simulink model "etc_plant_tf"  (R2022b)
settings: Solver=VariableStepAuto  StartTime=0.0  StopTime=20  RelTol=1e-3  EnableMultiTasking=on
PreLoadFcn:
  | % Throttle body parameters
  | etc_plant_data;
  | 
  | % Input data
  | load throttle_input;
values from neighbouring files (symbols this model uses):
  J = 2.45e-4    (= 0.000245)    [etc_plant_data.m]
  Kd = 0.03    [etc_plant_data.m]
  Km = 3.0    (= 3)    [etc_plant_data.m]
  Ks = 0.2    [etc_plant_data.m]
  theta_eq = pi/6    (= 0.523598775598)    [etc_plant_data.m]
settings Model: Creator=nicholas  LastModifiedBy=bensweet
settings SolverCC: ZeroCrossControl=EnableAll  AlgebraicLoopSolver=TrustRegion  AutoInsertRateTranBlk=on
settings DataIOCC: ExternalInput=[t, duty, direction]  LoadExternalInput=on  SaveState=on  ReturnWorkspaceOutputs=off
settings OptimizationCC: ExpressionDepthLimit=2147483647  InitFltsAndDblsToZero=on  LifeSpan=1  EfficientTunableParamExpr=on
settings DebuggingCC: UnconnectedInputMsg=warning  UnconnectedOutputMsg=warning  UnconnectedLineMsg=warning  PregeneratedLibrarySubsystemCodeDiagnostic=none  SFMachineParentedDataDiag=warning
settings HardwareCC: ProdBitPerPointer=32  ProdBitPerSizeT=32  ProdBitPerPtrDiffT=32  ProdLargestAtomicFloat=None  ProdIntDivRoundTo=Undefined  ProdEndianess=Unspecified  ProdWordSize=32  ProdHWDeviceType=32-bit Generic
settings ModelReferenceCC: EnableRefExpFcnMdlSchedulingChecks=on  PropagateSignalLabelsOutOfModel=off
settings SFSimCC: SimUseLocalCustomCode=off  MATLABDynamicMemAlloc=off
settings RTWCC: Description=RTW Embedded Coder (no auto configuration)  SystemTargetFile=ert.tlc  GenCodeOnly=on  TemplateMakefile=ert_default_tmf  RTWUseLocalCustomCode=off  DLArmComputeVersion=19.05
settings CodeAppCC: IgnoreCustomStorageClasses=off  CustomSymbolStrType=$N$R$M  StateflowObjectComments=on  InternalIdentifier=Classic
settings ERTTargetCC: TargetFcnLib=ansi_tfl_tmw.mat  MultiwordLength=2048  GenerateSampleERTMain=on  ERTCustomFileTemplate=example_file_process.tlc  ConvertIfToSwitch=off  SuppressUnreachableDefaultCases=off
settings ConfigComp: CovMetricSettings=dw  CovSaveCumulativeToWorkspaceVar=on  CovSaveSingleToWorkspaceVar=on  CovExternalEMLEnable=off  CovSFcnEnable=off

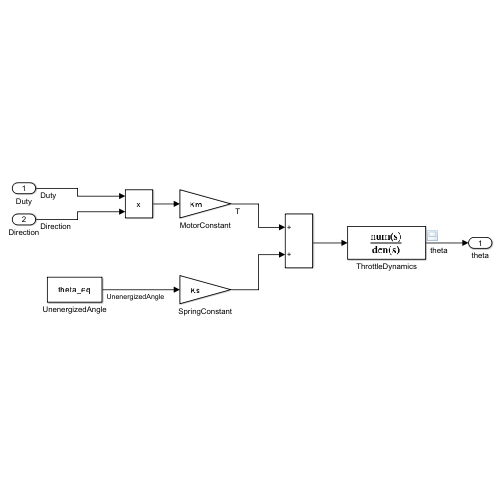
[thumbnail: Simulink's stored preview of the top-level diagram]
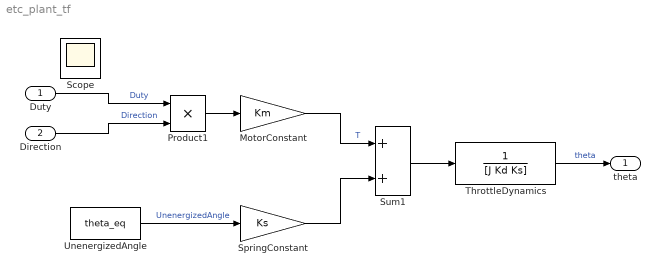
== system etc_plant_tf ==
  Duty : Inport
  Direction : Inport  Port=2
  MotorConstant : Gain  Gain=Km  SaturateOnIntegerOverflow=on  OutDataTypeStr=Inherit: Same as input  ParamDataTypeStr=Inherit: Same as input
  Product1 : Product  SaturateOnIntegerOverflow=on  OutDataTypeStr=Inherit: Same as first input
  SpringConstant : Gain  Gain=Ks  SaturateOnIntegerOverflow=on  OutDataTypeStr=Inherit: Same as input  ParamDataTypeStr=Inherit: Same as input
  Sum1 : Sum  SaturateOnIntegerOverflow=on
  ThrottleDynamics : TransferFcn  Denominator=[J Kd Ks]
  UnenergizedAngle : Constant  Value=theta_eq
  theta : Outport  VectorParamsAs1DForOutWhenUnconnected=off
  Scope : Scope
  wires:
  Product1/1 -> MotorConstant/1
  UnenergizedAngle/1 -> SpringConstant/1  "UnenergizedAngle"
  Duty/1 -> Product1/1  "Duty"
  Direction/1 -> Product1/2  "Direction"
  MotorConstant/1 -> Sum1/1  "T"
  SpringConstant/1 -> Sum1/2
  Sum1/1 -> ThrottleDynamics/1
  ThrottleDynamics/1 -> theta/1  "theta"
